simulink model "UnstablePlant"  (Simulink 9.0)
settings: Solver=VariableStepAuto  StartTime=0.0  StopTime=10.0  RelTol=1e-3
values from neighbouring files (symbols this model uses):
  Kp = 0.3    [open_loop.m]
  Ts = 0.005    [closed_loop.m]    (also in open_loop.m)
settings Model: Creator=tomas  LastModifiedBy=tomas
settings DataIOCC: SaveFormat=Dataset
settings OptimizationCC: LifeSpan=auto
settings DebuggingCC: UnderspecifiedInitializationDetection=Simplified  MergeDetectMultiDrivingBlocksExec=error  SFUnexpectedBacktrackingDiag=error  SFNoUnconditionalDefaultTransitionDiag=error  SFExecutionAtInitializationDiag=warning
settings HardwareCC: ProdBitPerPointer=64  ProdBitPerSizeT=64  ProdBitPerPtrDiffT=64  ProdLargestAtomicFloat=Float  ProdIntDivRoundTo=Zero  ProdEndianess=LittleEndian  ProdWordSize=64  ProdHWDeviceType=Intel->x86-64 (Windows64)
settings ModelReferenceCC: PropagateSignalLabelsOutOfModel=on
settings CodeAppCC: StateflowObjectComments=off
settings GRTTargetCC: TargetLangStandard=C99 (ISO)
settings ConfigComp: CovMetricSettings=dwe  CovHtmlReporting=off  CovSaveCumulativeToWorkspaceVar=off  CovSaveSingleToWorkspaceVar=off  CovExternalEMLEnable=on

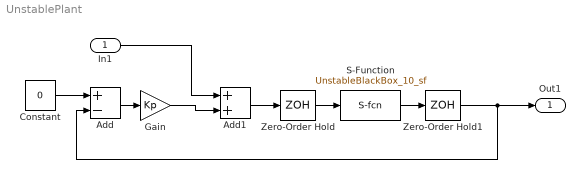
== system UnstablePlant ==
  In1 : Inport
  Add : Sum  Inputs=+-
  Add1 : Sum
  Constant : Constant  Value=0
  Gain : Gain  Gain=Kp
  S-Function : S-Function  FunctionName=UnstableBlackBox_10_sf  SFunctionDeploymentMode=off  EnableBusSupport=off  SFcnStateName=DWORK0
      settings: SFcnIsStateOwnerBlock=on
  Zero-Order Hold : ZeroOrderHold  SampleTime=Ts
  Zero-Order Hold1 : ZeroOrderHold  SampleTime=Ts
  Out1 : Outport
  wires:
  S-Function/1 -> Zero-Order Hold1/1
  Zero-Order Hold/1 -> S-Function/1
  In1/1 -> Add1/1
  Zero-Order Hold1/1 -> Add/2, Out1/1
  Constant/1 -> Add/1
  Add1/1 -> Zero-Order Hold/1
  Add/1 -> Gain/1
  Gain/1 -> Add1/2
